simulink model "IMPexample3sim"  (R2018a)
settings: Solver=VariableStepAuto  StartTime=0.0  StopTime=10.0  RelTol=1e-3
values from neighbouring files (symbols this model uses):
  Jp = acker(Ap',Cp',-100)'    [IMPexample2.m]    (also in IMPexample3.m)
  Jv = acker(Av',Cv',[-10 -10 -10 -10])'    [IMPexample2.m]    (also in IMPexample3.m = acker(Av',Cv',[-10 -10 -10])')
  Kp = acker(Ap,Bp,-10)    [IMPexample2.m]    (also in IMPexample3.m)
  Kpre = 1/evalfr(T,0)    [IMPexample2.m]    (also in IMPexample3.m)
  ref = 70*2*pi/60    (= 7.33038285838)    [IMPexample.m]    (also in IMPexample2.m; IMPexample3.m)
undefined symbols (not defined in the file or in its folder): Ap, Av, Bp, Cp, Cv
settings Model: Creator=Tobias Scala  LastModifiedBy=Tobias Scala

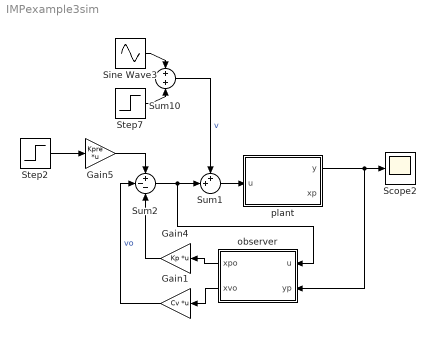
== system IMPexample3sim ==
  Gain1 : Gain  Gain=Cv  Multiplication=Matrix(K*u)
  Gain4 : Gain  Gain=Kp  Multiplication=Matrix(K*u)
  Gain5 : Gain  Gain=Kpre  Multiplication=Matrix(K*u)
  Scope2 : Scope
  Sine Wave3 : Sin  Amplitude=2  Frequency=2*ref  SampleTime=0
  Step2 : Step  After=ref  SampleTime=0
  Step7 : Step  Time=4  After=2  SampleTime=0
  Sum1 : Sum  Inputs=++|
  Sum10 : Sum  Inputs=+|+
  Sum2 : Sum  Inputs=+--
  observer : Subsystem
  plant : Subsystem
  wires:
  Sine Wave3/1 -> Sum10/1
  observer/2(xvo) -> Gain1/1
  Step7/1 -> Sum10/2
  plant/1(y) -> observer/2(yp), Scope2/1
  Sum10/1 -> Sum1/1  "v"
  Step2/1 -> Gain5/1
  Sum1/1 -> plant/1(u)
  Gain1/1 -> Sum2/2  "vo"
  Sum2/1 -> Sum1/2, observer/1(u)
  observer/1(xpo) -> Gain4/1
  Gain5/1 -> Sum2/1
  Gain4/1 -> Sum2/3

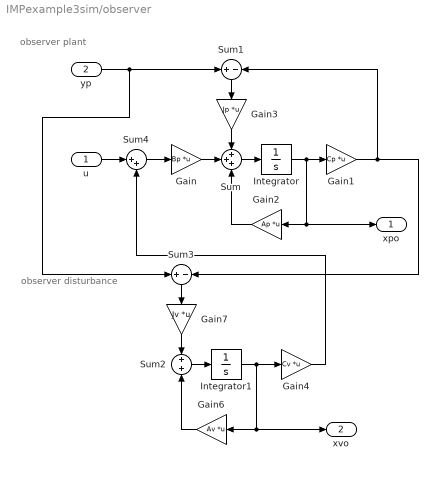
== system IMPexample3sim/observer ==
  note: observer disturbance
  note: observer plant
  u : Inport
  yp : Inport  Port=2
  Gain : Gain  Gain=Bp  Multiplication=Matrix(K*u)
  Gain1 : Gain  Gain=Cp  Multiplication=Matrix(K*u)
  Gain2 : Gain  Gain=Ap  Multiplication=Matrix(K*u)
  Gain3 : Gain  Gain=Jp  Multiplication=Matrix(K*u)
  Gain4 : Gain  Gain=Cv  Multiplication=Matrix(K*u)
  Gain6 : Gain  Gain=Av  Multiplication=Matrix(K*u)
  Gain7 : Gain  Gain=Jv  Multiplication=Matrix(K*u)
  Integrator : Integrator
  Integrator1 : Integrator
  Sum : Sum  Inputs=+++
  Sum1 : Sum  Inputs=+|-
  Sum2 : Sum  Inputs=+|+
  Sum3 : Sum  Inputs=+|-
  Sum4 : Sum  Inputs=|++
  xpo : Outport
  xvo : Outport  Port=2
  wires:
  Gain1/1 -> Sum3/2, Sum1/2
  u/1 -> Sum4/1
  Sum/1 -> Integrator/1
  Integrator/1 -> xpo/1, Gain2/1, Gain1/1
  Gain/1 -> Sum/2
  Gain2/1 -> Sum/3
  Sum1/1 -> Gain3/1
  Gain3/1 -> Sum/1
  yp/1 -> Sum3/1, Sum1/1
  Sum3/1 -> Gain7/1
  Gain6/1 -> Sum2/2
  Sum2/1 -> Integrator1/1
  Gain7/1 -> Sum2/1
  Integrator1/1 -> Gain4/1, xvo/1, Gain6/1
  Sum4/1 -> Gain/1
  Gain4/1 -> Sum4/2

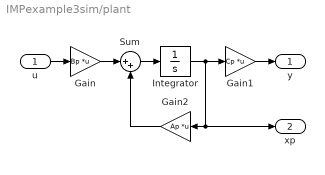
== system IMPexample3sim/plant ==
  u : Inport
  Gain : Gain  Gain=Bp  Multiplication=Matrix(K*u)
  Gain1 : Gain  Gain=Cp  Multiplication=Matrix(K*u)
  Gain2 : Gain  Gain=Ap  Multiplication=Matrix(K*u)
  Integrator : Integrator
  Sum : Sum  Inputs=|++
  y : Outport
  xp : Outport  Port=2
  wires:
  Gain1/1 -> y/1
  Gain/1 -> Sum/1
  Gain2/1 -> Sum/2
  u/1 -> Gain/1
  Sum/1 -> Integrator/1
  Integrator/1 -> xp/1, Gain2/1, Gain1/1
